simulink model "Positive_power_measurement"  (R2014b)
settings: Solver=ode45  StartTime=0.0  StopTime=10.0  RelTol=1e-3
undefined symbols (not defined in the file or in its folder): Pbase, Ts, Vline_rms_high, Vline_rms_low
libraries: powerlib_extras x2
settings Model: Creator=anony  LastModifiedBy=anony

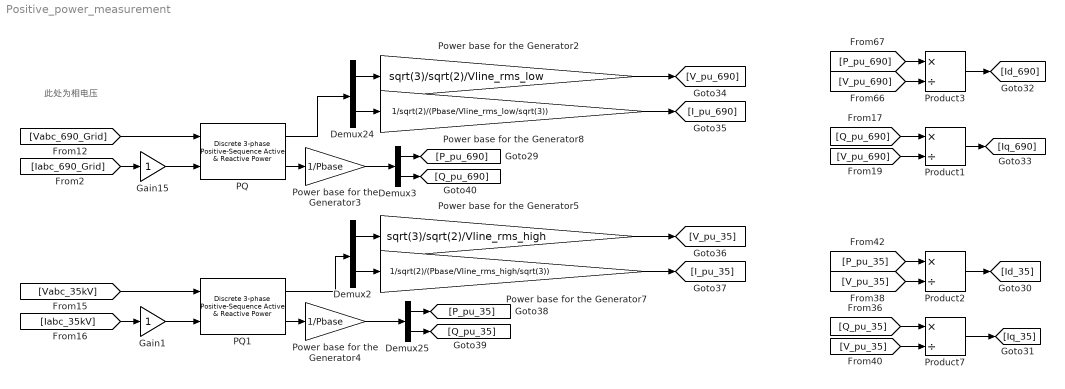
== system Positive_power_measurement ==
  note: 此处为相电压
  Demux{2..3,24..25} (4 alike) : Demux  Outputs=2
  Gain1 : Gain
  Gain15 : Gain
  PQ : powerlib_extras/Discrete Measurements/Discrete 3-phase  Positive-Sequence  Active & Reactive Power  Freq=Fnom  Par_Vinit=[0 0]  Par_Iinit=[0 0]  Ts=Ts
  PQ1 : powerlib_extras/Discrete Measurements/Discrete 3-phase  Positive-Sequence  Active & Reactive Power  Freq=Fnom  Par_Vinit=[0 0]  Par_Iinit=[0 0]  Ts=Ts
  Power base for the Generator2 : Gain  Gain=sqrt(3)/sqrt(2)/Vline_rms_low  SaturateOnIntegerOverflow=on  OutDataTypeStr=Inherit: Same as input  ParamDataTypeStr=Inherit: Same as input
  Power base for the Generator3 : Gain  Gain=1/Pbase  SaturateOnIntegerOverflow=on  OutDataTypeStr=Inherit: Same as input  ParamDataTypeStr=Inherit: Same as input
  Power base for the Generator4 : Gain  Gain=1/Pbase  SaturateOnIntegerOverflow=on  OutDataTypeStr=Inherit: Same as input  ParamDataTypeStr=Inherit: Same as input
  Power base for the Generator5 : Gain  Gain=sqrt(3)/sqrt(2)/Vline_rms_high  SaturateOnIntegerOverflow=on  OutDataTypeStr=Inherit: Same as input  ParamDataTypeStr=Inherit: Same as input
  Power base for the Generator7 : Gain  Gain=1/sqrt(2)/(Pbase/Vline_rms_high/sqrt(3))  SaturateOnIntegerOverflow=on  OutDataTypeStr=Inherit: Same as input  ParamDataTypeStr=Inherit: Same as input
  Power base for the Generator8 : Gain  Gain=1/sqrt(2)/(Pbase/Vline_rms_low/sqrt(3))  SaturateOnIntegerOverflow=on  OutDataTypeStr=Inherit: Same as input  ParamDataTypeStr=Inherit: Same as input
  Product{1..3,7} (4 alike) : Product  Inputs=*/  RndMeth=Zero
  wires:
  [Vabc_690_Grid] -> PQ/1
  [Iabc_690_Grid] -> Gain15/1
  PQ/2 -> Power base for the Generator3/1
  Gain15/1 -> PQ/2
  [Vabc_35kV] -> PQ1/1
  [Iabc_35kV] -> Gain1/1
  PQ1/2 -> Power base for the Generator4/1
  Gain1/1 -> PQ1/2
  [Q_pu_35] -> Product7/1
  [V_pu_35] -> Product7/2
  [P_pu_35] -> Product2/1
  [V_pu_35] -> Product2/2
  Product2/1 -> [Id_35]
  Product7/1 -> [Iq_35]
  [Q_pu_690] -> Product1/1
  [V_pu_690] -> Product1/2
  Product1/1 -> [Iq_690]
  [P_pu_690] -> Product3/1
  [V_pu_690] -> Product3/2
  Product3/1 -> [Id_690]
  Demux24/1 -> Power base for the Generator2/1
  Demux24/2 -> Power base for the Generator8/1
  Power base for the Generator8/1 -> [I_pu_690]
  Power base for the Generator2/1 -> [V_pu_690]
  PQ/1 -> Demux24/1
  Power base for the Generator3/1 -> Demux3/1
  Demux2/1 -> Power base for the Generator5/1
  Demux2/2 -> Power base for the Generator7/1
  Power base for the Generator7/1 -> [I_pu_35]
  Power base for the Generator5/1 -> [V_pu_35]
  PQ1/1 -> Demux2/1
  Demux25/1 -> [P_pu_35]
  Demux25/2 -> [Q_pu_35]
  Power base for the Generator4/1 -> Demux25/1
  Demux3/1 -> [P_pu_690]
  Demux3/2 -> [Q_pu_690]
